simulink model "Ex9_8model"  (R2013a)
settings: Solver=ode45  StartTime=0.0  StopTime=2  FixedStep=.001  RelTol=1e-3
settings Model: Creator=John  LastModifiedBy=John
settings DataIOCC: SignalLoggingSaveFormat=ModelDataLogs
settings OptimizationCC: ExpressionDepthLimit=2147483647
settings DebuggingCC: FcnCallInpInsideContextMsg=UseLocalSettings  StrictBusMsg=Warning
settings GRTTargetCC: CombineOutputUpdateFcns=off  GRTInterface=on

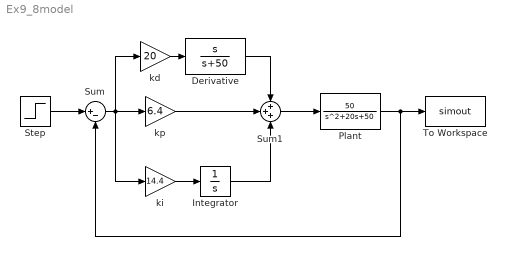
== system Ex9_8model ==
  "Derivative " : TransferFcn  Numerator=[1 0]  Denominator="[1  50]"
  Integrator : Integrator
  Plant : TransferFcn  Numerator=[50]  Denominator=[1 20 50]
  Step : Step  Time=.1  SampleTime=0
  Sum : Sum  Inputs=|+-
  Sum1 : Sum  Inputs=+++
  To Workspace : ToWorkspace  VariableName=simout  SampleTime=-1
  kd : Gain  Gain=20
  ki : Gain  Gain=14.4
  kp : Gain  Gain=6.4
  wires:
  Plant/1 -> To Workspace/1, Sum/2
  Sum/1 -> kp/1, ki/1, kd/1
  Step/1 -> Sum/1
  ki/1 -> Integrator/1
  Sum1/1 -> Plant/1
  kp/1 -> Sum1/2
  Integrator/1 -> Sum1/3
  kd/1 -> "Derivative "/1
  "Derivative "/1 -> Sum1/1
